simulink model "mrsObjectTrackingModel"  (R2024b)
settings: Solver=VariableStepAuto  StartTime=0.0  StopTime=inf  FixedStep=0.01  RelTol=1e-3  EnableMultiTasking=on
PreLoadFcn:
  | % Simulation parameters
  | load exampleMap
  | sampleTime = 0.05;
  | 
  | % Object Detector parameters
  | objX = 4;
  | objY = 4;
  | targetLabel = 1;
  | objLabel = 1;
  | objDetectorOffset = [0 0];
  | objDetectorAngle = 0;
  | objDetectorFOV = pi/3;
  | objDetectorRange = 5;
  | objDetectorColors = [1 0 0;0 1 0;0 0 1];
  | objDetectorMaxHits = 3;
libraries: mobileRoboticsLib x4
settings Model: Creator=scastro  LastModifiedBy=Matthew
settings SolverCC: AlgebraicLoopSolver=TrustRegion
settings DataIOCC: LimitDataPoints=on  ReturnWorkspaceOutputs=off
settings OptimizationCC: LifeSpan=inf
settings DebuggingCC: UnconnectedInputMsg=warning  UnconnectedOutputMsg=warning  UnconnectedLineMsg=warning  AllowSymbolicDim=off  SFUnexpectedBacktrackingDiag=warning  SFNoUnconditionalDefaultTransitionDiag=warning  SFExecutionAtInitializationDiag=none  ArithmeticOperatorsInVariantConditions=warning
settings ModelReferenceCC: EnableRefExpFcnMdlSchedulingChecks=on
settings SFSimCC: SimUseLocalCustomCode=off  CustomCodeUndefinedFunction=UseInterfaceOnly
settings RTWCC: RTWUseLocalCustomCode=off  GPUComputeCapability=3.5
settings CodeAppCC: StateflowObjectComments=on
settings GRTTargetCC: TargetLangStandard=C89/C90 (ANSI)
settings ConfigComp: CovMetricSettings=dw  CovSaveCumulativeToWorkspaceVar=on  CovSaveSingleToWorkspaceVar=on  CovExternalEMLEnable=off  CovSFcnEnable=off
settings SimscapeCC: SimscapeNominalValues="[{\"value\":\"10\",\"unit\":\"V\"},{\"value\":\"1\",\"unit\":\"A\"},{\"value\":\"10\",\"unit\":\"N*m\"},{\"value\":\"10\",\"unit\":\"bar\"},{\"value\":\"100\",\"unit\":\"kJ/kg\"},{\"value\":\"1\",\"unit\":\"kW\"},{\"value\":\"300\",\"unit\":\"K\"},{\"value\":\"100\",\"unit\":\"cm^3/s\"},{\"value\":\"1\",\"unit\":\"kN\"},{\"value\":\"1\",\"unit\":\"g/cm^3\"},{\"value\":\"1\",\"unit\":\"l\"},{\"value\":\"1\",\"unit\":\"cm^2\"},{\"value\":\"60\",\"unit\":\"Hz\"}]"  SimscapeLogType=all  SimscapeLogDataHistory=10000
settings ConfigurationSet: Description=SimMechanics 2G
settings ExplorerConfigSet: InternalSimMechanicsExplorerSettings="<ExplorerConfiguration><canonicalview>default</canonicalview><AnimationSetting><BasePlaybackSpeed>1.0</BasePlaybackSpeed><PlaybackSpeedFactor>1.0</PlaybackSpeedFactor></AnimationSetting><TilePanel><TileInfo><Tiles Columns=\"1\" Count=\"1\" Rows=\"1\"><Column Weight=\"1\"/><Row Weight=\"1\"/><Tile Height=\"1\" Width=\"1\" X=\"0\" Y=\"0\"/></Tiles></TileInfo><SceneInfo><SceneViewer><BGColor><R>0.60000002384185791</R><G>0.60000002384185791</G><B>0.60000002384185791</B></BGColor><Camera><DoPerspective>off</DoPerspective><Position><X>-1.70656042355848525</X><Y>-0.974920623359631922</Y><Z>4.72930454537082046</Z></Position><Center><X>0.552860638431633689</X><Y>1.42025063411503494</Y><Z>1.4843509506914252</Z></Center><Up><X>0.664249622453917166</X><Y>0.300615402055903091</Y><Z>0.684399604848363485</Z></Up><ViewLimDist>1</ViewLimDist><YLim>2.77881717169207398</YLim><XLim>3.55928742670435394</XLim></Camera></SceneViewer></SceneInfo></TilePanel><MechEditorPanel><Cameras/><GfxPanelCameraMap/><VideoCreator><PlaybackSpeedRatio>1.0</PlaybackSpeedRatio><FrameRate>30</FrameRate><VideoFormat>Motion JPEG AVI</VideoFormat><FrameSize>auto</FrameSize></VideoCreator></MechEditorPanel></ExplorerConfiguration>"

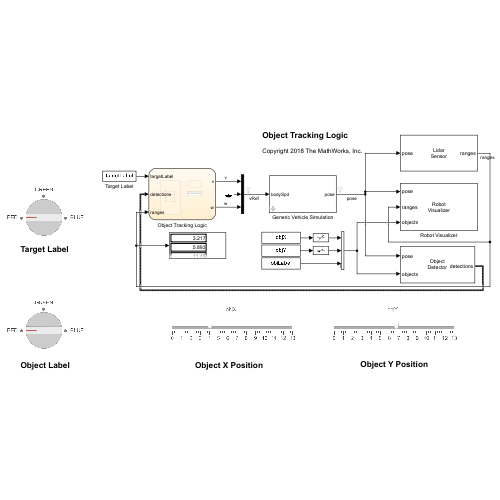
[thumbnail: Simulink's stored preview of the top-level diagram]
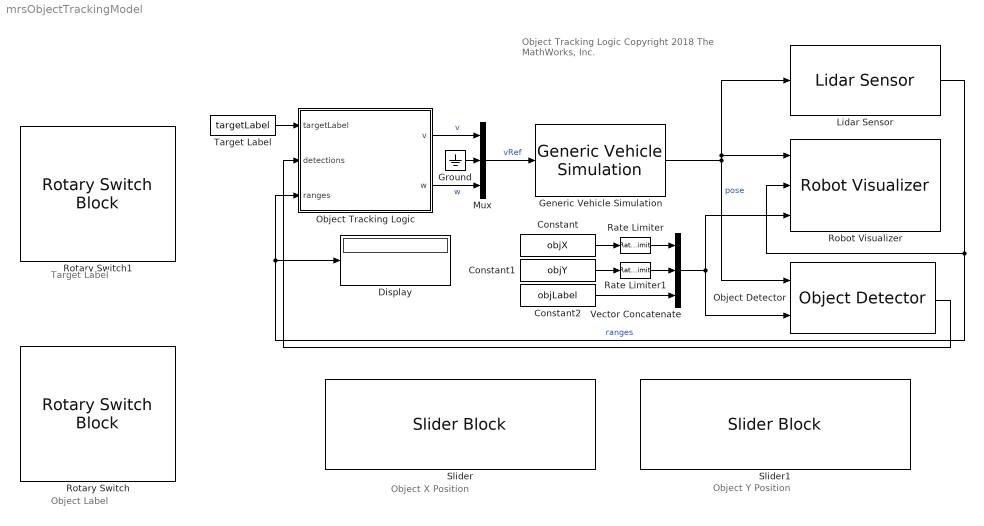
== system mrsObjectTrackingModel ==
  note: Target Label
  note: Object X Position
  note: Object Y Position
  note: Object Label
  note: Object Tracking Logic
      |
      | Copyright 2018 The MathWorks, Inc.
  Constant : Constant  Value=objX
  Constant1 : Constant  Value=objY
  Constant2 : Constant  Value=objLabel
  Display : Display
  Generic Vehicle Simulation : mobileRoboticsLib/Utilities/Generic Vehicle Simulation  initX=2  initY=3  initAngle=0  Ts=sampleTime
      settings: SourceProductName=Mobile Robotics Simulation Library
  Ground : Ground
  Lidar Sensor : mobileRoboticsLib/Environments/Lidar Sensor  mapName=map  sensorOffset=sensorOffset  scanAngles=[2, 1.5, 0]  maxRange=600
      settings: SourceProductName=Ground Vehicles Library
  Mux : Mux  Inputs=3
  Object Detector : mobileRoboticsLib/Environments/Object Detector  mapName=map  sensorOffset=objDetectorOffset  sensorAngle=objDetectorAngle  fieldOfView=objDetectorFOV  maxRange=objDetectorRange  maxDetections=objDetectorMaxHits  sampleTime=-1
      settings: SourceProductName=Ground Vehicles Library
  Object Tracking Logic : Stateflow chart  TreatAsAtomicUnit=on
  Rate Limiter : RateLimiter  SampleTimeMode=inherited  InitialCondition=objX
  Rate Limiter1 : RateLimiter  SampleTimeMode=inherited  InitialCondition=objX
  Robot Visualizer : mobileRoboticsLib/Environments/Robot Visualizer  Priority=99  robotRadius=0  mapName=map  showTrajectory=on  hasWaypoints=off  hasLidar=on  sensorOffset=[ 0 0 ]  scanAngles=[2, 1.5, 0]  hasObjDetector=on  objDetectorOffset=objDetectorOffset  objDetectorAngle=objDetectorAngle  objDetectorFOV=objDetectorFOV  objDetectorMaxRange=objDetectorRange  objectColors=objDetectorColors  objectMarkers=s
      settings: SourceProductName=Ground Vehicles Library
  Rotary Switch : RotarySwitchBlock  LabelPosition=Hide
      settings: Values={{'RED', 'GREEN', 'BLUE'}, [1 2 3]}
  Rotary Switch1 : RotarySwitchBlock  LabelPosition=Hide
      settings: Values={{'RED', 'GREEN', 'BLUE'}, [1 2 3]}
  Slider : SliderBlock  ScaleMax=13
  Slider1 : SliderBlock  ScaleMax=13
  Target Label : Constant  Value=targetLabel
  Vector Concatenate : Concatenate  NumInputs=3  Mode=Multidimensional array  ConcatenateDimension=2
  wires:
  Generic Vehicle Simulation/1 -> Lidar Sensor/1, Robot Visualizer/1, Object Detector/1  "pose"
  Object Tracking Logic/2(w) -> Mux/3  "w"
  Mux/1 -> Generic Vehicle Simulation/1  "vRef"
  Object Tracking Logic/1(v) -> Mux/1  "v"
  Object Detector/1 -> Object Tracking Logic/2(detections)
  Vector Concatenate/1 -> Robot Visualizer/3, Object Detector/2
  Constant/1 -> Rate Limiter/1
  Constant1/1 -> Rate Limiter1/1
  Constant2/1 -> Vector Concatenate/3
  Rate Limiter/1 -> Vector Concatenate/1
  Rate Limiter1/1 -> Vector Concatenate/2
  Target Label/1 -> Object Tracking Logic/1(targetLabel)
  Ground/1 -> Mux/2
  Lidar Sensor/1 -> Object Tracking Logic/3(ranges), Display/1, Robot Visualizer/2  "ranges"

== stateflow chart mrsObjectTrackingModel/Object Tracking Logic ==
  state TrackObject
    entry, during:
    [range,angle,valid] = findValidObject(targetLabel);
    if valid
    count = 0;
    else
    count = count + 1;
    end
    (default) -> (junction 20)
    TrackObject -> (junction 20) [order 1]
    (junction 20) -> (junction 24) [order 1] : % Set angular speed if
        | % angle outside deadband
        | [abs(angle) > pi/24]
    (junction 20) -> (junction 30) [order 2] : {w = 0;}
    (junction 24) -> (junction 49) : % Proportional
        | % control
        | {w = 1.5*angle;}
    (junction 49) -> (junction 30)
    (junction 30) -> (junction 54)
    (junction 54) -> (junction 56) [order 1] : % Go forward if object is far
        | [range > 1]
    (junction 54) -> (junction 60) [order 2] : {v = 0;}
    (junction 56) -> (junction 58) : {v = 0.5*range;}
    (junction 58) -> (junction 60)
  state SeekObject
    entry, during:
    v = 0.5;
    if (ranges(1) > ranges(2) || ranges(3) < 1)
    w = -2;
    else
    w = 2;
    end
  (default) -> TrackObject : {
      | count = 0;
      | range = 0;
      | angle = 0;
      | }
  TrackObject -> SeekObject [order 1] : [count > 20]
  SeekObject -> TrackObject : [~isempty(detections)]
  data: dist function_output; ang function_output; flag function_output; label function_input; targetLabel input; detections input size=[objDetectorMaxHits,3]; v output; w output; angle local; range local; count local; valid local; ranges input size=3
  function [dist,ang,flag] = findValidObject(label):
    | function [dist,ang,flag] = findValidObject(label)
    | % Finds the distance (dist) and angle (ang) of the nearest valid
    | % object detected. If an object is found, the (flag) output is true.
    | 
    | % Initialize
    | flag = false;
    | dist = 0;
    | ang = 0;
    | 
    | if ~isempty(detections)
    |     % Loop through all detections
    |     for idx = 1:size(detections,1)
    |         % If a detection matching the target label is found, 
    |         % return it and set the valid flag to true.
    |         if detections(idx,3) == label
    |             dist = detections(idx,1);
    |             ang  = detections(idx,2);
    |             flag = true;
    |             return; 
    |         end
    |     end
    | end
